simulink model "TestXformPL_example"  (R2017a)
settings: Solver=ode3  StartTime=0.0  StopTime=1000  FixedStep=1  RelTol=1e-3  EnableMultiTasking=on
libraries: Lib_PF_LineAC_TMATS x3, Lib_PF_BusLoadAC_TMATS x3, Lib_PF_BusGenAC_TMATS x1, Lib_Solve_SSNRSolverJC_TMATS x1, Lib_PF_BusSlackAC_TMATS x1, Lib_PF_XformerBAC_TMATS x1
settings Model: Creator=jwchapm2  LastModifiedBy=glthoma1
settings DataIOCC: LimitDataPoints=on  SaveFormat=Array
settings OptimizationCC: LifeSpan=inf
settings DebuggingCC: SFUnexpectedBacktrackingDiag=warning  SFNoUnconditionalDefaultTransitionDiag=warning  SFExecutionAtInitializationDiag=none
settings HardwareCC: ProdBitPerPointer=32  ProdBitPerSizeT=32  ProdBitPerPtrDiffT=32  ProdLargestAtomicFloat=None  ProdIntDivRoundTo=Undefined  ProdEndianess=Unspecified  ProdWordSize=32  ProdHWDeviceType=32-bit Generic
settings ModelReferenceCC: PropagateSignalLabelsOutOfModel=off
settings GRTTargetCC: TargetLangStandard=C89/C90 (ANSI)  GeneratePreprocessorConditionals=Disable all
settings ConfigComp: CovMetricSettings=dw  CovHtmlReporting=on  CovSaveCumulativeToWorkspaceVar=on  CovSaveSingleToWorkspaceVar=on  CovExternalEMLEnable=off

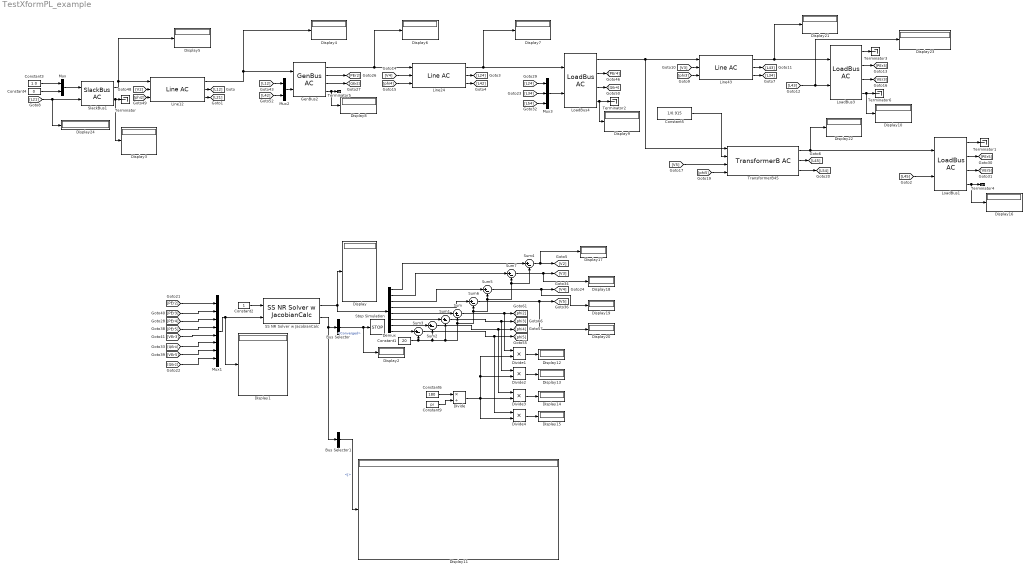
== system TestXformPL_example ==
  Bus Selector : BusSelector  OutputSignals=Converged
  Bus Selector1 : BusSelector  OutputSignals=J
  Constant1 : Constant  Value=20
  Constant2 : Constant
  Constant3 : Constant  Value=1.0
  Constant4 : Constant  Value=0
  Constant5 : Constant  Value=1/0.915
  Constant6 : Constant  Value=180
  Constant9 : Constant  Value=pi
  Demux : Demux  Outputs=8
  Display{,1..24} (25 alike) : Display
  Divide : Product  Inputs=*/
  Divide{1..4} (4 alike) : Product  Inputs=**
  GenBus2 : Lib_PF_BusGenAC_TMATS/GenBus AC  PeInEN_M=off  BlkNm_M=double(gcb)  Vispec_M=1.0  P_M=1.5  Qmax_M=1000  Qmin_M=-1000
  Line12 : Lib_PF_LineAC_TMATS/Line AC  R_M=0.001  X_M=0.05  Z2R_M=0  Z2X_M=-20
  Line24 : Lib_PF_LineAC_TMATS/Line AC  R_M=0.001  X_M=0.05  Z2R_M=0  Z2X_M=-20
  Line43 : Lib_PF_LineAC_TMATS/Line AC  R_M=0.001  X_M=0.05  Z2R_M=0  Z2X_M=-20
  LoadBus1 : Lib_PF_BusLoadAC_TMATS/LoadBus AC  PeInEN_M=off  P_M=-1  QeInEN_M=off  Q_M=-0.5  BlkNm_M=double(gcb)
  LoadBus3 : Lib_PF_BusLoadAC_TMATS/LoadBus AC  PeInEN_M=off  P_M=-0.5  QeInEN_M=off  Q_M=-0.1  BlkNm_M=double(gcb)
  LoadBus4 : Lib_PF_BusLoadAC_TMATS/LoadBus AC  PeInEN_M=off  P_M=0  QeInEN_M=off  Q_M=0  BlkNm_M=double(gcb)
  Mux : Mux  Inputs=2
  Mux1 : Mux  Inputs=8
  Mux2 : Mux  Inputs=2
  Mux3 : Mux  Inputs=3
  SS NR Solver w JacobianCalc : Lib_Solve_SSNRSolverJC_TMATS/SS NR Solver w JacobianCalc  SJac_Per_M=[0.01,0.01,0.01,0.01,0.01,0.01,0.01,0.01;-0.01,-0.01,-0.01,-0.01,-0.01,-0.01,-0.01,-0.01]  SNR_IC_M=[21 21 21 21 20 20 20 20]  SNR_DX_M=5  SNR_Mx_M=100000  SNR_Mn_M=0.00000001  SJacobianAttempts_M=20  Cond_Limits_M=0.00000001
  SlackBus1 : Lib_PF_BusSlackAC_TMATS/SlackBus AC
  Stop Simulation : Stop
  Sum{,1..7} (8 alike) : Sum  Inputs=|+-
  Terminator{,1..6} (7 alike) : Terminator
  TransformerB45 : Lib_PF_XformerBAC_TMATS/TransformerB AC  R_M=0  X_M=0.1  alpha_M=0  b_M=1
  wires:
  SlackBus1/1 -> Line12/1, Display5/1
  Line12/1 -> GenBus2/1, Display4/1
  SlackBus1/2 -> Display3/1, Terminator/1
  SS NR Solver w JacobianCalc/2 -> Bus Selector1/1, Bus Selector/1
  Bus Selector/1 -> Display2/1, Stop Simulation/1  "<Converged>"
  Mux1/1 -> Display1/1, SS NR Solver w JacobianCalc/2
  Constant2/1 -> SS NR Solver w JacobianCalc/1
  SS NR Solver w JacobianCalc/1 -> Demux/1, Display/1
  Line24/3 -> [L42]
  [V4] -> Line24/2
  [phi4] -> Line24/3
  GenBus2/1 -> Line24/1, Display6/1
  Line24/1 -> LoadBus4/1, Display7/1
  [L45] -> LoadBus1/2
  LoadBus1/2 -> [PEr5]
  LoadBus1/3 -> [VEr5]
  Line24/2 -> [L24]
  Constant3/1 -> Mux/1
  Constant4/1 -> Mux/2
  Mux/1 -> SlackBus1/1
  GenBus2/2 -> [PEr2]
  GenBus2/3 -> [QEr2]
  Demux/5 -> Sum/1
  Constant1/1 -> Sum4/2, Sum7/2, Sum5/2, Sum6/2, Sum/2, Sum1/2, Sum2/2, Sum3/2
  Sum/1 -> Divide1/1, [phi2]
  Demux/6 -> Sum1/1
  Demux/7 -> Sum2/1
  Demux/8 -> Sum3/1
  Sum3/1 -> Divide4/1, [phi5]
  Sum2/1 -> Divide3/1, [phi4]
  Sum1/1 -> Divide2/1, [phi3]
  Bus Selector1/1 -> Display11/1  "<J>"
  Line12/2 -> [L12]
  Line12/3 -> [L21]
  [phi2] -> Line12/3
  Mux2/1 -> GenBus2/2
  [L12] -> Mux2/1
  [L42] -> Mux2/2
  LoadBus4/1 -> TransformerB45/1, Line43/1
  [V5] -> TransformerB45/3
  [phi5] -> TransformerB45/4
  TransformerB45/1 -> LoadBus1/1, Display22/1
  TransformerB45/2 -> [L45]
  Mux3/1 -> LoadBus4/2
  [L34] -> Mux3/2
  [L24] -> Mux3/1
  [L54] -> Mux3/3
  LoadBus1/4 -> Display16/1, Terminator4/1
  GenBus2/4 -> Display8/1, Terminator5/1
  LoadBus4/2 -> [PEr4]
  LoadBus4/3 -> [QEr4]
  Constant5/1 -> TransformerB45/2
  [V2] -> Line12/2
  Divide1/1 -> Display12/1
  Constant6/1 -> Divide/1
  Constant9/1 -> Divide/2
  Divide/1 -> Divide4/2, Divide3/2, Divide2/2, Divide1/2
  Divide2/1 -> Display13/1
  Divide3/1 -> Display14/1
  Divide4/1 -> Display15/1
  LoadBus1/1 -> Terminator1/1
  LoadBus4/4 -> Display9/1, Terminator2/1
  Line43/3 -> [L34]
  [V3] -> Line43/2
  [phi3] -> Line43/3
  Line43/1 -> LoadBus3/1, Display21/1
  Line43/2 -> [L43]
  [L43] -> LoadBus3/2, Display23/1
  LoadBus3/1 -> Terminator3/1
  LoadBus3/2 -> [PEr3]
  LoadBus3/3 -> [VEr3]
  LoadBus3/4 -> Display10/1, Terminator6/1
  Demux/1 -> Sum4/1
  Demux/2 -> Sum7/1
  Demux/3 -> Sum5/1
  Demux/4 -> Sum6/1
  [PEr2] -> Mux1/1
  [PEr4] -> Mux1/3
  [PEr3] -> Mux1/2
  [PEr5] -> Mux1/4
  [QEr4] -> Mux1/6
  [VEr5] -> Mux1/7
  [QEr2] -> Mux1/8
  [VEr3] -> Mux1/5
  Sum6/1 -> Display20/1, [V5]
  Sum7/1 -> Display18/1, [V3]
  Sum5/1 -> Display19/1, [V4]
  Sum4/1 -> Display17/1, [V2]
  [L21] -> SlackBus1/2, Display24/1
  TransformerB45/3 -> [L54]
